simulink model "verify_reward"  (R2025b)
settings: Solver=ode4  StartTime=0.0  StopTime=8.5  FixedStep=0.01  RelTol=1e-5  AbsTol=1e-6
libraries: sldvlib x7
settings Model: Creator=Deermste  LastModifiedBy=Deermste
settings ConfigComp: DVMode=DesignErrorDetection  DVMaxProcessTime=300.0  DVMaxTestCaseSteps=10000.0  DVTestSuiteOptimization=Auto  DVAbsoluteTolerance=1.0e-5  DVDefectChecker=on  DVDetectOutOfBounds=on  DVMaxViolationSteps=20.0  DVModelReferenceHarness=on  DVHarnessSource=Signal Editor  DVActiveTab=0.0

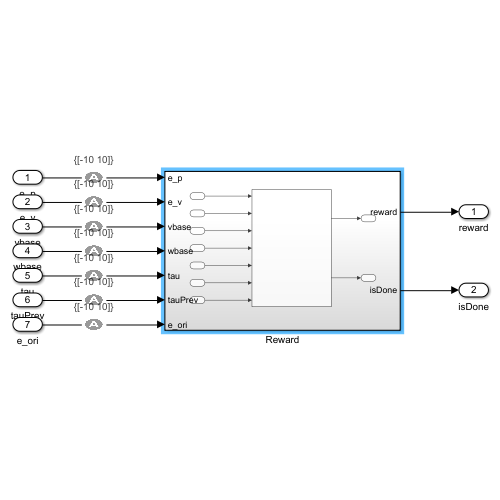
[thumbnail: Simulink's stored preview of the top-level diagram]
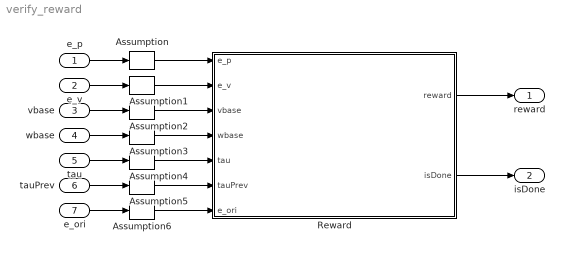
== system verify_reward ==
  e_p : Inport  OutMin=[-10]  OutMax=[10]
  e_v : Inport  Port=2  OutMin=[-10]  OutMax=[10]
  vbase : Inport  Port=3  OutMin=[-10]  OutMax=[10]
  wbase : Inport  Port=4  OutMin=[-10]  OutMax=[10]
  tau : Inport  Port=5  OutMin=[-10]  OutMax=[10]
  tauPrev : Inport  Port=6  OutMin=[-10]  OutMax=[10]
  e_ori : Inport  Port=7  OutMin=[-10]  OutMax=[10]
  Assumption{,1..6} (7 alike) : sldvlib/Objectives and Constraints/Assumption  enabled=on  customAVTBlockType=Assumption  intervals={[-10 10]}  initial=off  dispValues=on  outEnabled=on
      settings: AttributesFormatString=%<intervals>
  Reward : Subsystem
  reward : Outport
  isDone : Outport  Port=2
  wires:
  e_p/1 -> Assumption/1
  e_v/1 -> Assumption1/1
  vbase/1 -> Assumption2/1
  wbase/1 -> Assumption3/1
  tau/1 -> Assumption4/1
  tauPrev/1 -> Assumption5/1
  e_ori/1 -> Assumption6/1
  Reward/1(reward) -> reward/1
  Reward/2(isDone) -> isDone/1
  Assumption/1 -> Reward/1(e_p)
  Assumption1/1 -> Reward/2(e_v)
  Assumption2/1 -> Reward/3(vbase)
  Assumption3/1 -> Reward/4(wbase)
  Assumption4/1 -> Reward/5(tau)
  Assumption5/1 -> Reward/6(tauPrev)
  Assumption6/1 -> Reward/7(e_ori)

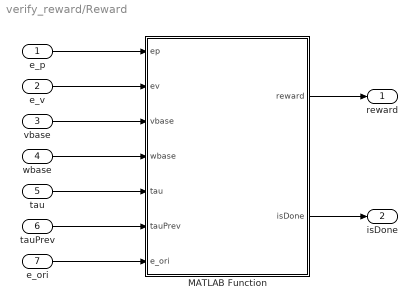
== system verify_reward/Reward ==
  e_p : Inport
  e_v : Inport  Port=2
  vbase : Inport  Port=3
  wbase : Inport  Port=4
  tau : Inport  Port=5
  tauPrev : Inport  Port=6
  e_ori : Inport  Port=7
  MATLAB Function : MATLAB Function  TreatAsAtomicUnit=on
  reward : Outport
  isDone : Outport  Port=2
  wires:
  MATLAB Function/1(reward) -> reward/1
  MATLAB Function/2(isDone) -> isDone/1
  e_ori/1 -> MATLAB Function/7(e_ori)
  e_p/1 -> MATLAB Function/1(ep)
  e_v/1 -> MATLAB Function/2(ev)
  vbase/1 -> MATLAB Function/3(vbase)
  wbase/1 -> MATLAB Function/4(wbase)
  tau/1 -> MATLAB Function/5(tau)
  tauPrev/1 -> MATLAB Function/6(tauPrev)

== matlab function verify_reward/Reward/MATLAB Function ==
  data: ep input; reward output; ev input; vbase input; wbase input; tau input; tauPrev input; isDone output; e_ori input
function [reward,isDone] = rewardFcn(ep, ev, vbase, wbase, tau, tauPrev, e_ori)
persistent prev_dist;
if isempty(prev_dist), prev_dist = inf; end
% if resetFlag     % <-- NEU
%     prev_dist = inf;
% end

% --- Frühcheck auf Finite ---
if any(~isfinite([ep;ev;vbase;wbase;e_ori;tau;tauPrev]))
    reward = -1; isDone = true; prev_dist = inf; return;
end

% ---- Gewichte (Startwerte) ----
W.wp   = 150;    % EE-Position
W.wv   = 25;     % EE-Geschwindigkeit
W.wori = 200;    % Basis-Orientierung (P)
W.wwb  = 8;      % Basis-Winkelgeschw. (D)
W.wvb  = 2;      % Basis-Linear
W.wu   = 0.02;   % Momente
W.wd   = 0.06;   % Delta-Momente (etwas höher für Smoothness)

% ---- Fortschritt ----
dist = norm(ep);
prog = 0;
if isfinite(prev_dist)
    d = prev_dist - dist;
    if d>0, prog = 10*d; end
end
prev_dist = dist;

% ---- Kosten ----
cost  = 0;
cost  = cost + W.wp  * (ep.'*ep);
cost  = cost + W.wv  * (ev.'*ev);
cost  = cost + W.wori* (e_ori.'*e_ori);  % << P auf Orientierung
cost  = cost + W.wwb * (wbase.'*wbase);  % << D auf Orientierung
cost  = cost + W.wvb * (vbase.'*vbase);
cost  = cost + W.wu  * (tau.'*tau);
cost  = cost + W.wd  * ((tau - tauPrev).'*(tau - tauPrev));

% Bonus nahe Bahnpunkt
bonus = 0.05 * exp( - (dist/0.02)^2 );

reward = (prog + bonus) - cost;
reward = reward / 500;

% Abbruch
isDone = false;
if isnan(reward) || ~all(isfinite([ep;ev;vbase;wbase;e_ori;tau;tauPrev])) || dist>10
    isDone = true; reward = -1; prev_dist = inf;
end
end
